simulink model "PV_MPPT_C2000_Algorithm"  (R2018b)
settings: Solver=FixedStepDiscrete  StartTime=0.0  StopTime=inf  FixedStep=1e-4  RelTol=1e-3  EnableMultiTasking=on
InitFcn:
  | IQ8 = 256;
  | IQ13 = 8192;
  | IQ15 = 32768;
  | IQ24 = 16777216;
  | 
  | InvFreq = 50;
  | 
  | Tdata = 0.05;
  | Tcontrol = 1e-4;
undefined symbols (not defined in the file): DiscIntNeverNeededParam, Down, GPTRIP1SEL, GPTRIP2SEL, TZ1, TZ2, Up
libraries: c2802xlib x8, simulink x4, c280xlib x3
settings Model: ExtModeTrigDuration=8  Creator=The MathWorks, Inc.  LastModifiedBy=jlesage
settings DataIOCC: LimitDataPoints=on  SaveFormat=Array  SaveOutput=off  SaveTime=off  SignalLoggingName=sigsOut
settings OptimizationCC: DefaultUnderspecifiedDataType=single  ExpressionDepthLimit=2147483647  InitFltsAndDblsToZero=on  LifeSpan=1  MaxStackSize=512
settings DebuggingCC: UnderspecifiedInitializationDetection=Classic  MergeDetectMultiDrivingBlocksExec=none  CheckExecutionContextPreStartOutputMsg=on  CheckExecutionContextRuntimeOutputMsg=on  SignalResolutionControl=TryResolveAllWithWarning  MultiTaskDSMMsg=warning  MultiTaskCondExecSysMsg=none  SigSpecEnsureSampleTimeMsg=none  FcnCallInpInsideContextMsg=warning  AllowSymbolicDim=off  StateNameClashWarn=warning  LibraryContextMissingDiagnostic=none  SFUnexpectedBacktrackingDiag=warning  SFNoUnconditionalDefaultTransitionDiag=warning  SFExecutionAtInitializationDiag=none
settings HardwareCC: ProdBitPerChar=16  ProdBitPerInt=16  ProdBitPerPointer=32  ProdBitPerSizeT=32  ProdBitPerPtrDiffT=32  ProdLargestAtomicInteger=Integer  ProdLargestAtomicFloat=None  ProdWordSize=16  ProdLongLongMode=on  ProdHWDeviceType=Texas Instruments->C2000  TargetBitPerChar=16  TargetBitPerInt=16  TargetBitPerPointer=16  TargetLargestAtomicInteger=Integer  TargetIntDivRoundTo=Zero  TargetEndianess=LittleEndian  TargetWordSize=16  TargetHWDeviceType=Texas Instruments->C2000  ProdEqTarget=off
settings ModelReferenceCC: UpdateModelReferenceTargets=IfOutOfDate  PropagateSignalLabelsOutOfModel=off
settings SFSimCC: SimUseLocalCustomCode=off
settings RTWCC: SystemTargetFile=ert.tlc  HardwareBoard=TI Piccolo F2803x  TemplateMakefile=ert_default_tmf  PostCodeGenCommand=; codertarget.postCodeGenHookCommand(h)  RTWUseLocalCustomCode=off  Toolchain=Texas Instruments Code Composer Studio (C2000)
settings CodeAppCC: IgnoreCustomStorageClasses=off  CustomSymbolStrType=$N$R$M  StateflowObjectComments=on  InternalIdentifier=Classic
settings ERTTargetCC: CodeReplacementLibrary=TI C28x  MultiwordLength=2048  ParMdlRefBuildCompliant=off  CompOptLevelCompliant=off  ConcurrentExecutionCompliant=off  SupportNonFinite=off  SupportComplex=off  CPPClassGenCompliant=off  ExtModeStaticAllocSize=2048  ConvertIfToSwitch=off  SuppressUnreachableDefaultCases=off
settings ConfigComp: CovMetricSettings=dw  CovHtmlReporting=on  CovSaveCumulativeToWorkspaceVar=on  CovSaveSingleToWorkspaceVar=on  CovExternalEMLEnable=off  CovSFcnEnable=off

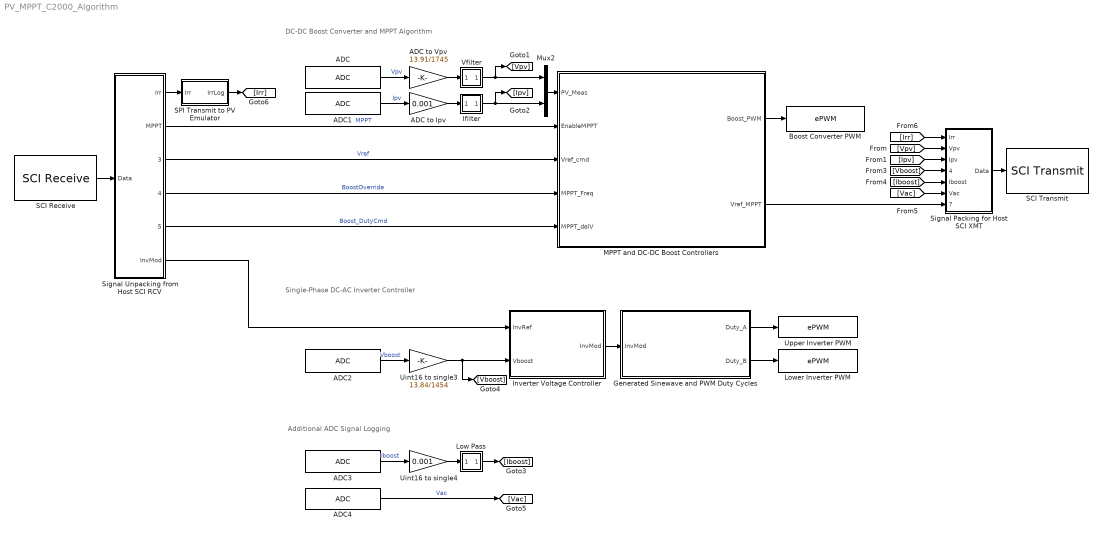
== system PV_MPPT_C2000_Algorithm ==
  note: Additional ADC Signal Logging
  note: Single-Phase DC-AC Inverter Controller
  note: DC-DC Boost Converter and MPPT Algorithm
  ADC : c2802xlib/ADC  ADCModule=1  samplingMode=Single sample mode  ADCResolution=12-bit (Single-ended input)  useSOC1=SOC0  useSOC2=SOC0_SOC1  SOCAcquisitionWindow=7  SOCTriggerSource=Software  SOCInterruptTrigger=No ADCINT  Ts=Tcontrol  dType=uint16  postInterrupt=off  interruptSel=ADCINT1  ADCINTContinuous=off  endma=off  chdma=1  blkParamProc=C2000  conv1=ADCINA1  conv2=ADCINA0 and ADCINB0  conv1_Type4=ADCIN0  conv2_Type4=ADCIN0 and ADCIN1
      settings: SourceProductName=Embedded Coder Support Package for Texas Instruments C2000 Processors
  ADC to Ipv : Gain  Gain=0.001  OutDataTypeStr=single
  ADC to Vpv : Gain  Gain=13.91/1745  OutDataTypeStr=single
  ADC1 : c2802xlib/ADC  ADCModule=1  samplingMode=Single sample mode  ADCResolution=12-bit (Single-ended input)  useSOC1=SOC1  useSOC2=SOC0_SOC1  SOCAcquisitionWindow=7  SOCTriggerSource=Software  SOCInterruptTrigger=No ADCINT  Ts=Tcontrol  dType=uint16  postInterrupt=off  interruptSel=ADCINT1  ADCINTContinuous=off  endma=off  chdma=1  blkParamProc=C2000  conv1=ADCINA0  conv2=ADCINA0 and ADCINB0  conv1_Type4=ADCIN0  conv2_Type4=ADCIN0 and ADCIN1
      settings: SourceProductName=Embedded Coder Support Package for Texas Instruments C2000 Processors
  ADC2 : c2802xlib/ADC  ADCModule=1  samplingMode=Single sample mode  ADCResolution=12-bit (Single-ended input)  useSOC1=SOC2  useSOC2=SOC0_SOC1  SOCAcquisitionWindow=7  SOCTriggerSource=Software  SOCInterruptTrigger=No ADCINT  Ts=Tcontrol  dType=uint16  postInterrupt=off  interruptSel=ADCINT1  ADCINTContinuous=off  endma=off  chdma=1  blkParamProc=C2000  conv1=ADCINA2  conv2=ADCINA0 and ADCINB0  conv1_Type4=ADCIN0  conv2_Type4=ADCIN0 and ADCIN1
      settings: SourceProductName=Embedded Coder Support Package for Texas Instruments C2000 Processors
  ADC3 : c2802xlib/ADC  ADCModule=1  samplingMode=Single sample mode  ADCResolution=12-bit (Single-ended input)  useSOC1=SOC3  useSOC2=SOC0_SOC1  SOCAcquisitionWindow=7  SOCTriggerSource=Software  SOCInterruptTrigger=No ADCINT  Ts=Tcontrol  dType=uint16  postInterrupt=off  interruptSel=ADCINT1  ADCINTContinuous=off  endma=off  chdma=1  blkParamProc=C2000  conv1=ADCINB6  conv2=ADCINA0 and ADCINB0  conv1_Type4=ADCIN0  conv2_Type4=ADCIN0 and ADCIN1
      settings: SourceProductName=Embedded Coder Support Package for Texas Instruments C2000 Processors
  ADC4 : c2802xlib/ADC  ADCModule=1  samplingMode=Single sample mode  ADCResolution=12-bit (Single-ended input)  useSOC1=SOC4  useSOC2=SOC0_SOC1  SOCAcquisitionWindow=7  SOCTriggerSource=Software  SOCInterruptTrigger=No ADCINT  Ts=Tcontrol  dType=uint16  postInterrupt=off  interruptSel=ADCINT1  ADCINTContinuous=off  endma=off  chdma=1  blkParamProc=C2000  conv1=ADCINA7  conv2=ADCINA0 and ADCINB0  conv1_Type4=ADCIN0  conv2_Type4=ADCIN0 and ADCIN1
      settings: SourceProductName=Embedded Coder Support Package for Texas Instruments C2000 Processors
  Boost Converter PWM : c2802xlib/ePWM  useModule=ePWM3  ePWMxLINKTBPRD=Not Linked  periodUnits=Clock cycles  timerSource=Specify via dialog  timerPeriod_clk=1500  timerPeriod_sec=0.0001  tbshadow=Counter equals to zero  countingMode=Up-Down  phaseActiveEnable=Set counter to phase value specified via dialog  phaseDirection=Count up after sync  phaseActive=4  synchronizationEnable=off  dcaevt1Sync=off  dcbevt1Sync=off  synchronizationOption=Disable  clockPrescale=1  HSclockPrescale=1  enswap=off  ePWMxAStatus=on  ePWMxAactionLogic1=Do nothing  ePWMxAactionLogic2=Do nothing  ePWMxAactionLogic3=Set  ePWMxAactionLogic4=Clear  ePWMxAactionLogic5=Do nothing  ePWMxAactionLogic6=Do nothing  ePWMxALoadMode=Load on counter equals to zero (CTR=Zero)  ePWMxACSFenable=off  ePWMxACSFvalue=Forcing disable  ePWMxASFreload=Zero  ePWMxBStatus=off  ePWMxBactionLogic1=Do nothing  ePWMxBactionLogic2=Do nothing  ePWMxBactionLogic3=Do nothing  ePWMxBactionLogic4=Do nothing  ePWMxBactionLogic5=Do nothing  ePWMxBactionLogic6=Do nothing  ePWMxBLoadMode=Load on counter equals to zero (CTR=Zero)  ePWMxBCSFenable=off  ePWMxBCSFvalue=Forcing disable  ePWMxBSFreload=Zero  ePWNxBOutWay=off  ePWMxLINKCMPA=Not Linked  CMPAUnits=Clock cycles  CMPASource=Input port  CMPAValue_per=0  CMPAValue_clk=0  enCMPAshadow=Counter equals to zero  ePWMxLINKCMPB=Not Linked  CMPBUnits=Clock cycles  CMPBSource=Specify via dialog  CMPBValue_per=50  CMPBValue_clk=0  enCMPBshadow=Counter equals to zero  ePWMxLINKCMPC=Not Linked  CMPCUnits=Clock cycles  CMPCSource=Specify via dialog  CMPCValue_per=50  CMPCValue_clk=32000  enCMPCshadow=Counter equals to zero  ePWMxLINKCMPD=Not Linked  CMPDUnits=Clock cycles  CMPDSource=Specify via dialog  CMPDValue_per=50  CMPDValue_clk=32000  enCMPDshadow=Counter equals to zero  enableDBePWMxA=on  enableDBePWMxB=on  enhalfcycle=off  DBpolarity=Active high (AH)  DBedgeDelay=Positive  DBSource_ePWMxA=ePWMxA  DBSource_ePWMxB=ePWMxA  DBperiodSource=Specify via dialog  REDperiod=0  FEDperiod=30  adcstartModuleA=on  adcrequestEventA=Second event  adcstartEventA=Counter is incrementing and equals to the compare B register (CTRU=CMPB)  adcstartEventA_type2=Digital Compare Module A Event 1 start of conversion (DCAEVT1.soc)  adcstartModuleB=off  adcrequestEventB=First event  adcstartEventB=Counter equals to zero (CTR=Zero)  adcstartEventB_type2=Counter equals to zero (CTR=Zero)  intEn=on  intPrd=Second event  intSel=Counter equals to period (CTR=PRD)  intSel_type2=Counter equals to zero (CTR=Zero)  hrpe=off  enHRPWM=off  HRPWM_LoadMode=Counter equals to period (CTR=PRD)  HRPWM_CTLMode=Duty or Period control mode  HRPWM_EDGMode=Falling edge  hrpeb=off  enHRPWMB=off  HRPWM_LoadModeB=Counter equals to zero (CTR=ZERO)  HRPWM_CTLModeB=Duty or Period control mode  HRPWM_EDGModeB=Both edge  enSFO=off  enautoconv=off  chopperEnable=off  chopperFrequency=1  chopperFirstwidth=1  chopperDuty=12.5%  tripZonesource=Specify via dialog  tzselOSHT1=off  tzselOSHT2=off  tzselOSHT3=off  tzselOSHDCAEV1=on  tzselOSHDCBEV1=off  tzselCBC1=off  tzselCBC2=off  tzselCBC3=off  tzselCBCDCAEV2=on  tzselCBCDCBEV2=off  tzselOSHT4=off  tzselOSHT5=off  tzselOSHT6=off  tzselCBC4=off  tzselCBC5=off  tzselCBC6=off  enTzOstIntr=off  enTzCbcIntr=off  enTzDCAEVT1Intr=off  enTzDCAEVT2Intr=off  enTzDCBEVT1Intr=off  enTzDCBEVT2Intr=off  ePWMxAforced=Low  ePWMxBforced=No action  DCAEVT1forced=No action  DCBEVT1forced=No action  DCAEVT2forced=No action  DCBEVT2forced=No action  dcah=COMP1OUT input  dcal=Trip Zone 2 input (TZ2)  dcbh=Trip Zone 1 input (TZ1)  dcbl=Trip Zone 2 input (TZ2)  dcah_type2=GPTRIP1SEL/(TZ1)  dcal_type2=GPTRIP2SEL/(TZ2)  dcbh_type2=GPTRIP1SEL/(TZ1)  dcbl_type2=GPTRIP2SEL/(TZ2)  gendcaevt1=DCAH=high and DCAL=don't care  gendcaevt2=Event disabled  gendcbevt1=Event disabled  gendcbevt2=Event disabled  dcaevt1src=DCAEVT1 with async  dcaevt2src=DCAEVT2 with sync  dcbevt1src=DCBEVT1 with sync  dcbevt2src=DCBEVT2 with sync  pulsesel=Counter equals to zero (CTR=Zero)  blankinv=off  blankoffset=0  blankwidth=0  evsrcsel=Filtered version of DCAEVT1 (DCAEVT1FILT)  encape=off  PwmType=C2000
      settings: SourceProductName=Embedded Coder Support Package for Texas Instruments C2000 Processors
  Generated Sinewave and PWM Duty Cycles : Subsystem
  Ifilter : Subsystem  mask{Tf=0.01}
      mask prompts: Tf "Filter Time Constant"
  Inverter Voltage Controller : Subsystem
  Low Pass : Subsystem  mask{Tf=0.01}
      mask prompts: Tf "Filter Time Constant"
  Lower Inverter PWM : c2802xlib/ePWM  useModule=ePWM2  ePWMxLINKTBPRD=Not Linked  periodUnits=Clock cycles  timerSource=Specify via dialog  timerPeriod_clk=1500  timerPeriod_sec=0.0001  tbshadow=Counter equals to zero  countingMode=Up-Down  phaseActiveEnable=Set counter to phase value specified via dialog  phaseDirection=Count up after sync  phaseActive=2  synchronizationEnable=off  dcaevt1Sync=off  dcbevt1Sync=off  synchronizationOption=Counter equals to zero (CTR=Zero)  clockPrescale=1  HSclockPrescale=1  enswap=off  ePWMxAStatus=on  ePWMxAactionLogic1=Do nothing  ePWMxAactionLogic2=Do nothing  ePWMxAactionLogic3=Clear  ePWMxAactionLogic4=Set  ePWMxAactionLogic5=Do nothing  ePWMxAactionLogic6=Do nothing  ePWMxALoadMode=Load on counter equals to period (CTR=PRD)  ePWMxACSFenable=off  ePWMxACSFvalue=Forcing disable  ePWMxASFreload=Zero  ePWMxBStatus=off  ePWMxBactionLogic1=Do nothing  ePWMxBactionLogic2=Do nothing  ePWMxBactionLogic3=Do nothing  ePWMxBactionLogic4=Do nothing  ePWMxBactionLogic5=Do nothing  ePWMxBactionLogic6=Do nothing  ePWMxBLoadMode=Load on counter equals to zero (CTR=Zero)  ePWMxBCSFenable=off  ePWMxBCSFvalue=Forcing disable  ePWMxBSFreload=Zero  ePWNxBOutWay=on  ePWMxLINKCMPA=Not Linked  CMPAUnits=Clock cycles  CMPASource=Input port  CMPAValue_per=0  CMPAValue_clk=750  enCMPAshadow=Counter equals to zero  ePWMxLINKCMPB=Not Linked  CMPBUnits=Clock cycles  CMPBSource=Specify via dialog  CMPBValue_per=50  CMPBValue_clk=0  enCMPBshadow=Counter equals to zero  ePWMxLINKCMPC=Not Linked  CMPCUnits=Clock cycles  CMPCSource=Specify via dialog  CMPCValue_per=50  CMPCValue_clk=32000  enCMPCshadow=Counter equals to zero  ePWMxLINKCMPD=Not Linked  CMPDUnits=Clock cycles  CMPDSource=Specify via dialog  CMPDValue_per=50  CMPDValue_clk=32000  enCMPDshadow=Counter equals to zero  enableDBePWMxA=on  enableDBePWMxB=on  enhalfcycle=off  DBpolarity=Active high complementary (AHC)  DBedgeDelay=Positive  DBSource_ePWMxA=ePWMxA  DBSource_ePWMxB=ePWMxB  DBperiodSource=Specify via dialog  REDperiod=20  FEDperiod=20  adcstartModuleA=on  adcrequestEventA=First event  adcstartEventA=Counter equals to zero (CTR=Zero)  adcstartEventA_type2=Digital Compare Module A Event 1 start of conversion (DCAEVT1.soc)  adcstartModuleB=off  adcrequestEventB=First event  adcstartEventB=Counter equals to zero (CTR=Zero)  adcstartEventB_type2=Counter equals to zero (CTR=Zero)  intEn=off  intPrd=First event  intSel=Counter equals to period (CTR=PRD)  intSel_type2=Counter equals to zero (CTR=Zero)  hrpe=off  enHRPWM=off  HRPWM_LoadMode=Counter equals to period (CTR=PRD)  HRPWM_CTLMode=Duty or Period control mode  HRPWM_EDGMode=Falling edge  hrpeb=off  enHRPWMB=off  HRPWM_LoadModeB=Counter equals to zero (CTR=ZERO)  HRPWM_CTLModeB=Duty or Period control mode  HRPWM_EDGModeB=Both edge  enSFO=off  enautoconv=off  chopperEnable=off  chopperFrequency=1  chopperFirstwidth=1  chopperDuty=12.5%  tripZonesource=Specify via dialog  tzselOSHT1=off  tzselOSHT2=off  tzselOSHT3=off  tzselOSHDCAEV1=on  tzselOSHDCBEV1=off  tzselCBC1=off  tzselCBC2=off  tzselCBC3=off  tzselCBCDCAEV2=on  tzselCBCDCBEV2=off  tzselOSHT4=off  tzselOSHT5=off  tzselOSHT6=off  tzselCBC4=off  tzselCBC5=off  tzselCBC6=off  enTzOstIntr=off  enTzCbcIntr=off  enTzDCAEVT1Intr=off  enTzDCAEVT2Intr=off  enTzDCBEVT1Intr=off  enTzDCBEVT2Intr=off  ePWMxAforced=Low  ePWMxBforced=No action  DCAEVT1forced=No action  DCBEVT1forced=No action  DCAEVT2forced=No action  DCBEVT2forced=No action  dcah=COMP1OUT input  dcal=Trip Zone 2 input (TZ2)  dcbh=Trip Zone 1 input (TZ1)  dcbl=Trip Zone 2 input (TZ2)  dcah_type2=GPTRIP1SEL/(TZ1)  dcal_type2=GPTRIP2SEL/(TZ2)  dcbh_type2=GPTRIP1SEL/(TZ1)  dcbl_type2=GPTRIP2SEL/(TZ2)  gendcaevt1=DCAH=high and DCAL=don't care  gendcaevt2=Event disabled  gendcbevt1=Event disabled  gendcbevt2=Event disabled  dcaevt1src=DCAEVT1 with async  dcaevt2src=DCAEVT2 with sync  dcbevt1src=DCBEVT1 with sync  dcbevt2src=DCBEVT2 with sync  pulsesel=Counter equals to zero (CTR=Zero)  blankinv=off  blankoffset=0  blankwidth=0  evsrcsel=Filtered version of DCAEVT1 (DCAEVT1FILT)  encape=off  PwmType=C2000
      settings: SourceProductName=Embedded Coder Support Package for Texas Instruments C2000 Processors
  MPPT and DC-DC Boost Controllers : Subsystem
  Mux2 : Mux  Inputs=2
  SCI Receive : c280xlib/SCI Receive  sciModule=A  dataHead='B'  dataTail='T'  dataType=uint16  dataDim=6  initValue=[0.1*IQ13 0.1*IQ13 25*IQ8 0.1*IQ13 0 3*IQ8]  errOption=Output the last received value  errValue=0.5*IQ13  sampleTime=Tdata  outputStatus=off  postInterrupt=off  numFifo=0
      settings: SourceProductName=Embedded Coder Support Package for Texas Instruments C2000 Processors  SourceProductBaseCode=TIC2000
  SCI Transmit : c280xlib/SCI Transmit  sciModule=A  dataHead='S'  dataTail='E'  postInterrupt=off  numFifo=0
      settings: SourceProductName=Embedded Coder Support Package for Texas Instruments C2000 Processors
  SPI Transmit to PV Emulator : Subsystem
  Signal Packing for Host SCI XMT : Subsystem
  Signal Unpacking from Host SCI RCV : Subsystem
  Uint16 to single3 : Gain  Gain=13.84/1454  OutDataTypeStr=single
  Uint16 to single4 : Gain  Gain=0.001  OutDataTypeStr=single
  Upper Inverter PWM : c2802xlib/ePWM  useModule=ePWM1  ePWMxLINKTBPRD=Not Linked  periodUnits=Clock cycles  timerSource=Specify via dialog  timerPeriod_clk=1500  timerPeriod_sec=0.0001  tbshadow=Counter equals to zero  countingMode=Up-Down  phaseActiveEnable=Disable  phaseDirection=Count down after sync  phaseActive=750  synchronizationEnable=off  dcaevt1Sync=off  dcbevt1Sync=off  synchronizationOption=Counter equals to zero (CTR=Zero)  clockPrescale=1  HSclockPrescale=1  enswap=off  ePWMxAStatus=on  ePWMxAactionLogic1=Do nothing  ePWMxAactionLogic2=Do nothing  ePWMxAactionLogic3=Clear  ePWMxAactionLogic4=Set  ePWMxAactionLogic5=Do nothing  ePWMxAactionLogic6=Do nothing  ePWMxALoadMode=Load on counter equals to zero (CTR=Zero)  ePWMxACSFenable=off  ePWMxACSFvalue=Forcing disable  ePWMxASFreload=Zero  ePWMxBStatus=off  ePWMxBactionLogic1=Do nothing  ePWMxBactionLogic2=Do nothing  ePWMxBactionLogic3=Do nothing  ePWMxBactionLogic4=Do nothing  ePWMxBactionLogic5=Do nothing  ePWMxBactionLogic6=Do nothing  ePWMxBLoadMode=Load on counter equals to zero (CTR=Zero)  ePWMxBCSFenable=off  ePWMxBCSFvalue=Forcing disable  ePWMxBSFreload=Zero  ePWNxBOutWay=on  ePWMxLINKCMPA=Not Linked  CMPAUnits=Clock cycles  CMPASource=Input port  CMPAValue_per=0  CMPAValue_clk=750  enCMPAshadow=Counter equals to zero  ePWMxLINKCMPB=Not Linked  CMPBUnits=Clock cycles  CMPBSource=Specify via dialog  CMPBValue_per=50  CMPBValue_clk=0  enCMPBshadow=Counter equals to zero  ePWMxLINKCMPC=Not Linked  CMPCUnits=Clock cycles  CMPCSource=Specify via dialog  CMPCValue_per=50  CMPCValue_clk=32000  enCMPCshadow=Counter equals to zero  ePWMxLINKCMPD=Not Linked  CMPDUnits=Clock cycles  CMPDSource=Specify via dialog  CMPDValue_per=50  CMPDValue_clk=32000  enCMPDshadow=Counter equals to zero  enableDBePWMxA=on  enableDBePWMxB=on  enhalfcycle=off  DBpolarity=Active high complementary (AHC)  DBedgeDelay=Positive  DBSource_ePWMxA=ePWMxA  DBSource_ePWMxB=ePWMxB  DBperiodSource=Specify via dialog  REDperiod=20  FEDperiod=20  adcstartModuleA=on  adcrequestEventA=First event  adcstartEventA=Counter equals to zero (CTR=Zero)  adcstartEventA_type2=Digital Compare Module A Event 1 start of conversion (DCAEVT1.soc)  adcstartModuleB=off  adcrequestEventB=First event  adcstartEventB=Counter equals to zero (CTR=Zero)  adcstartEventB_type2=Counter equals to zero (CTR=Zero)  intEn=off  intPrd=First event  intSel=Counter equals to period (CTR=PRD)  intSel_type2=Counter equals to zero (CTR=Zero)  hrpe=off  enHRPWM=off  HRPWM_LoadMode=Counter equals to period (CTR=PRD)  HRPWM_CTLMode=Duty or Period control mode  HRPWM_EDGMode=Falling edge  hrpeb=off  enHRPWMB=off  HRPWM_LoadModeB=Counter equals to zero (CTR=ZERO)  HRPWM_CTLModeB=Duty or Period control mode  HRPWM_EDGModeB=Both edge  enSFO=off  enautoconv=off  chopperEnable=off  chopperFrequency=1  chopperFirstwidth=1  chopperDuty=12.5%  tripZonesource=Specify via dialog  tzselOSHT1=off  tzselOSHT2=off  tzselOSHT3=off  tzselOSHDCAEV1=on  tzselOSHDCBEV1=off  tzselCBC1=off  tzselCBC2=off  tzselCBC3=off  tzselCBCDCAEV2=on  tzselCBCDCBEV2=off  tzselOSHT4=off  tzselOSHT5=off  tzselOSHT6=off  tzselCBC4=off  tzselCBC5=off  tzselCBC6=off  enTzOstIntr=off  enTzCbcIntr=off  enTzDCAEVT1Intr=off  enTzDCAEVT2Intr=off  enTzDCBEVT1Intr=off  enTzDCBEVT2Intr=off  ePWMxAforced=Low  ePWMxBforced=No action  DCAEVT1forced=No action  DCBEVT1forced=No action  DCAEVT2forced=No action  DCBEVT2forced=No action  dcah=COMP1OUT input  dcal=Trip Zone 2 input (TZ2)  dcbh=Trip Zone 1 input (TZ1)  dcbl=Trip Zone 2 input (TZ2)  dcah_type2=GPTRIP1SEL/(TZ1)  dcal_type2=GPTRIP2SEL/(TZ2)  dcbh_type2=GPTRIP1SEL/(TZ1)  dcbl_type2=GPTRIP2SEL/(TZ2)  gendcaevt1=DCAH=high and DCAL=don't care  gendcaevt2=Event disabled  gendcbevt1=Event disabled  gendcbevt2=Event disabled  dcaevt1src=DCAEVT1 with async  dcaevt2src=DCAEVT2 with sync  dcbevt1src=DCBEVT1 with sync  dcbevt2src=DCBEVT2 with sync  pulsesel=Counter equals to zero (CTR=Zero)  blankinv=off  blankoffset=0  blankwidth=0  evsrcsel=Filtered version of DCAEVT1 (DCAEVT1FILT)  encape=off  PwmType=C2000
      settings: SourceProductName=Embedded Coder Support Package for Texas Instruments C2000 Processors
  Vfilter : Subsystem  mask{Tf=0.01}
      mask prompts: Tf "Filter Time Constant"
  wires:
  ADC/1 -> ADC to Vpv/1  "Vpv"
  ADC1/1 -> ADC to Ipv/1  "Ipv"
  ADC2/1 -> Uint16 to single3/1  "Vboost"
  ADC3/1 -> Uint16 to single4/1  "Iboost"
  Generated Sinewave and PWM Duty Cycles/1(Duty_A) -> Upper Inverter PWM/1
  Generated Sinewave and PWM Duty Cycles/2(Duty_B) -> Lower Inverter PWM/1
  ADC to Vpv/1 -> Vfilter/1(u)
  ADC to Ipv/1 -> Ifilter/1(u)
  Uint16 to single4/1 -> Low Pass/1(u)
  ADC4/1 -> [Vac]  "Vac"
  MPPT and DC-DC Boost Controllers/1(Boost_PWM) -> Boost Converter PWM/1
  Mux2/1 -> MPPT and DC-DC Boost Controllers/1(PV_Meas)
  [Irr] -> Signal Packing for Host SCI XMT/1(Irr)
  [Vpv] -> Signal Packing for Host SCI XMT/2(Vpv)
  [Ipv] -> Signal Packing for Host SCI XMT/3(Ipv)
  [Vboost] -> Signal Packing for Host SCI XMT/4(Vboost)
  [Iboost] -> Signal Packing for Host SCI XMT/5(Iboost)
  [Vac] -> Signal Packing for Host SCI XMT/6(Vac)
  MPPT and DC-DC Boost Controllers/2(Vref_MPPT) -> Signal Packing for Host SCI XMT/7(Dboost)
  Signal Packing for Host SCI XMT/1(Data) -> SCI Transmit/1
  Signal Unpacking from Host SCI RCV/5(MPPT_Vinc) -> MPPT and DC-DC Boost Controllers/5(MPPT_delV)  "Boost_DutyCmd"
  Signal Unpacking from Host SCI RCV/4(MPPT_Freq) -> MPPT and DC-DC Boost Controllers/4(MPPT_Freq)  "BoostOverride"
  Signal Unpacking from Host SCI RCV/2(MPPT) -> MPPT and DC-DC Boost Controllers/2(EnableMPPT)  "MPPT"
  Signal Unpacking from Host SCI RCV/3(Vref_cmd) -> MPPT and DC-DC Boost Controllers/3(Vref_cmd)  "Vref"
  Uint16 to single3/1 -> [Vboost], Inverter Voltage Controller/2(Vboost)
  Signal Unpacking from Host SCI RCV/6(InvMod) -> Inverter Voltage Controller/1(InvRef)
  Inverter Voltage Controller/1(InvMod) -> Generated Sinewave and PWM Duty Cycles/1(InvMod)
  Signal Unpacking from Host SCI RCV/1(Irr) -> SPI Transmit to PV Emulator/1(Irr)
  SCI Receive/1 -> Signal Unpacking from Host SCI RCV/1(Data)
  SPI Transmit to PV Emulator/1(IrrLog) -> [Irr]
  Vfilter/1(y) -> Mux2/1, [Vpv]
  Ifilter/1(y) -> Mux2/2, [Ipv]
  Low Pass/1(y) -> [Iboost]

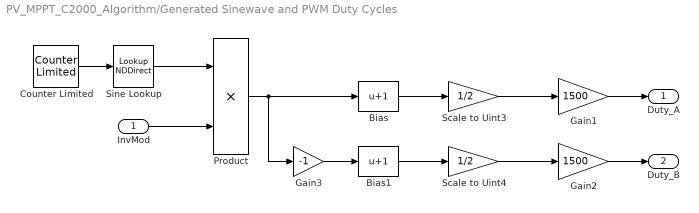
== system PV_MPPT_C2000_Algorithm/Generated Sinewave and PWM Duty Cycles ==
  InvMod : Inport
  Bias : Bias  Bias=1
  Bias1 : Bias  Bias=1
  Counter Limited : simulink/Sources/Counter Limited  uplimit=floor(1/(InvFreq*Tcontrol))  tsamp=Tcontrol
  Gain1 : Gain  Gain=1500  ParamDataTypeStr=uint16  OutDataTypeStr=uint16  RndMeth=Simplest
  Gain2 : Gain  Gain=1500  ParamDataTypeStr=uint16  OutDataTypeStr=uint16  RndMeth=Simplest
  Gain3 : Gain  Gain=-1
  Product : Product
  Scale to Uint3 : Gain  Gain=1/2  OutDataTypeStr=single
  Scale to Uint4 : Gain  Gain=1/2  OutDataTypeStr=single
  Sine Lookup : LookupNDDirect  NumberOfTableDimensions=1  Table=sin( 2*pi * (0:floor(1/(InvFreq*Tcontrol)))/floor(1/(InvFreq*Tcontrol))+90/180)'  TableDataTypeStr=single
  Duty_A : Outport
  Duty_B : Outport  Port=2
  wires:
  Bias/1 -> Scale to Uint3/1
  Scale to Uint4/1 -> Gain2/1
  InvMod/1 -> Product/2
  Bias1/1 -> Scale to Uint4/1
  Scale to Uint3/1 -> Gain1/1
  Product/1 -> Gain3/1, Bias/1
  Gain3/1 -> Bias1/1
  Sine Lookup/1 -> Product/1
  Counter Limited/1 -> Sine Lookup/1
  Gain1/1 -> Duty_A/1
  Gain2/1 -> Duty_B/1

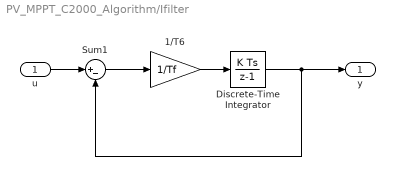
== system PV_MPPT_C2000_Algorithm/Ifilter ==
  u : Inport
  1/T6 : Gain  Gain=1/Tf
  Discrete-Time Integrator : DiscreteIntegrator  SampleTime=Tcontrol  ICPrevOutput=DiscIntNeverNeededParam  ICPrevScaledInput=DiscIntNeverNeededParam
  Sum1 : Sum  Inputs=|+-
  y : Outport
  wires:
  Sum1/1 -> 1/T6/1
  Discrete-Time Integrator/1 -> Sum1/2, y/1
  u/1 -> Sum1/1
  1/T6/1 -> Discrete-Time Integrator/1

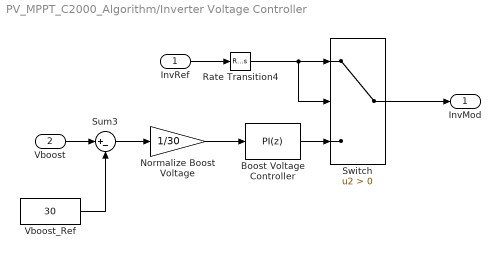
== system PV_MPPT_C2000_Algorithm/Inverter Voltage Controller ==
  InvRef : Inport
  Vboost : Inport  Port=2
  Boost Voltage Controller : simulink/Continuous/PID Controller  Controller=PI  TimeDomain=Discrete-time  SampleTime=Tcontrol  IntegratorMethod=Forward Euler  FilterMethod=Forward Euler  Form=Parallel  UseFilter=on  ControllerParametersSource=internal  P=3  I=250  D=0  N=100  InitialConditionSource=internal  InitialConditionForIntegrator=1  InitialConditionForFilter=0  ExternalReset=none  LimitOutput=on  UpperSaturationLimit=1  LowerSaturationLimit=0  LinearizeAsGain=on  AntiWindupMode=clamping  Kb=1  TrackingMode=off  Kt=1  PParamMin=[]  PParamMax=[]  IParamMin=[]  IParamMax=[]  DParamMin=[]  DParamMax=[]  NParamMin=[]  NParamMax=[]  KbParamMin=[]  KbParamMax=[]  KtParamMin=[]  KtParamMax=[]  POutMin=[]  POutMax=[]  IOutMin=[]  IOutMax=[]  DOutMin=[]  DOutMax=[]  NOutMin=[]  NOutMax=[]  KbOutMin=[]  KbOutMax=[]  KtOutMin=[]  KtOutMax=[]  IntegratorOutMin=[]  IntegratorOutMax=[]  FilterOutMin=[]  FilterOutMax=[]  SumOutMin=[]  SumOutMax=[]  SumI1OutMin=[]  SumI1OutMax=[]  SumI2OutMin=[]  SumI2OutMax=[]  SumI3OutMin=[]  SumI3OutMax=[]  SumDOutMin=[]  SumDOutMax=[]  SaturationOutMin=[]  SaturationOutMax=[]  IntegratorContinuousStateAttributes=''  IntegratorStateMustResolveToSignalObject=off  IntegratorRTWStateStorageClass=Auto  FilterContinuousStateAttributes=''  FilterStateMustResolveToSignalObject=off  FilterRTWStateStorageClass=Auto  DifferentiatorICPrevScaledInput=0  DifferentiatorOutMin=[]  DifferentiatorOutMax=[]  InitialConditionSetting=State (most efficient)  FilterDiffOutCoefMin=[]  FilterDiffOutCoefMax=[]  SumDenOutMin=[]  SumDenOutMax=[]  SumNumOutMin=[]  SumNumOutMax=[]  ReciprocalOutMin=[]  ReciprocalOutMax=[]  DivideOutMin=[]  DivideOutMax=[]  TunerSelectOption=Transfer Function Based (PID Tuner App)
  Normalize Boost Voltage : Gain  Gain=1/30
  Rate Transition4 : RateTransition  Integrity=off  Deterministic=off  InitialCondition=0.1*IQ24  OutPortSampleTime=Tcontrol
  Sum3 : Sum  Inputs=|+-
  Switch : Switch  Criteria=u2 > Threshold
  Vboost_Ref : Constant  Value=30  OutDataTypeStr=single
  InvMod : Outport
  wires:
  InvRef/1 -> Rate Transition4/1
  Rate Transition4/1 -> Switch/2, Switch/1
  Vboost_Ref/1 -> Sum3/2
  Sum3/1 -> Normalize Boost Voltage/1
  Normalize Boost Voltage/1 -> Boost Voltage Controller/1
  Switch/1 -> InvMod/1
  Boost Voltage Controller/1 -> Switch/3
  Vboost/1 -> Sum3/1

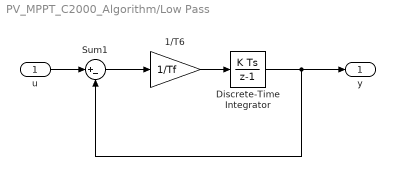
== system PV_MPPT_C2000_Algorithm/Low Pass ==
  u : Inport
  1/T6 : Gain  Gain=1/Tf
  Discrete-Time Integrator : DiscreteIntegrator  SampleTime=Tcontrol  ICPrevOutput=DiscIntNeverNeededParam  ICPrevScaledInput=DiscIntNeverNeededParam
  Sum1 : Sum  Inputs=|+-
  y : Outport
  wires:
  1/T6/1 -> Discrete-Time Integrator/1
  u/1 -> Sum1/1
  Discrete-Time Integrator/1 -> y/1, Sum1/2
  Sum1/1 -> 1/T6/1

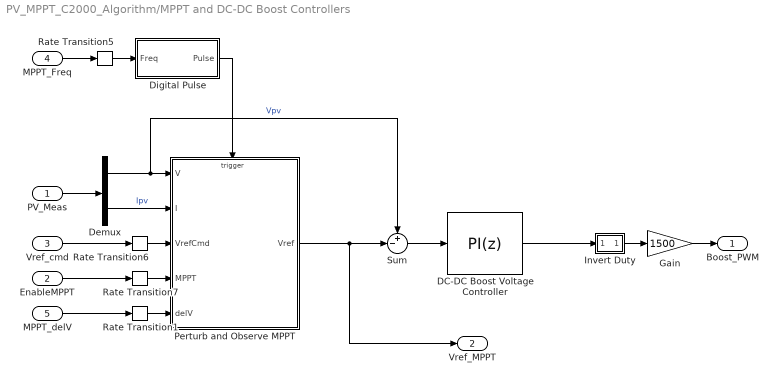
== system PV_MPPT_C2000_Algorithm/MPPT and DC-DC Boost Controllers ==
  PV_Meas : Inport
  EnableMPPT : Inport  Port=2
  Vref_cmd : Inport  Port=3
  MPPT_Freq : Inport  Port=4
  MPPT_delV : Inport  Port=5
  DC-DC Boost Voltage Controller : simulink/Continuous/PID Controller  Controller=PI  TimeDomain=Discrete-time  SampleTime=Tcontrol  IntegratorMethod=Forward Euler  FilterMethod=Forward Euler  Form=Parallel  UseFilter=on  ControllerParametersSource=internal  P=0.015  I=2.5  D=0  N=100  InitialConditionSource=internal  InitialConditionForIntegrator=0  InitialConditionForFilter=0  ExternalReset=none  LimitOutput=on  UpperSaturationLimit=0.9  LowerSaturationLimit=0  LinearizeAsGain=on  AntiWindupMode=clamping  Kb=1  TrackingMode=off  Kt=1  PParamMin=[]  PParamMax=[]  IParamMin=[]  IParamMax=[]  DParamMin=[]  DParamMax=[]  NParamMin=[]  NParamMax=[]  KbParamMin=[]  KbParamMax=[]  KtParamMin=[]  KtParamMax=[]  POutMin=[]  POutMax=[]  IOutMin=[]  IOutMax=[]  DOutMin=[]  DOutMax=[]  NOutMin=[]  NOutMax=[]  KbOutMin=[]  KbOutMax=[]  KtOutMin=[]  KtOutMax=[]  IntegratorOutMin=[]  IntegratorOutMax=[]  FilterOutMin=[]  FilterOutMax=[]  SumOutMin=[]  SumOutMax=[]  SumI1OutMin=[]  SumI1OutMax=[]  SumI2OutMin=[]  SumI2OutMax=[]  SumI3OutMin=[]  SumI3OutMax=[]  SumDOutMin=[]  SumDOutMax=[]  SaturationOutMin=[]  SaturationOutMax=[]  IntegratorContinuousStateAttributes=''  IntegratorStateMustResolveToSignalObject=off  IntegratorRTWStateStorageClass=Auto  FilterContinuousStateAttributes=''  FilterStateMustResolveToSignalObject=off  FilterRTWStateStorageClass=Auto  DifferentiatorICPrevScaledInput=0  DifferentiatorOutMin=[]  DifferentiatorOutMax=[]  InitialConditionSetting=State (most efficient)  FilterDiffOutCoefMin=[]  FilterDiffOutCoefMax=[]  SumDenOutMin=[]  SumDenOutMax=[]  SumNumOutMin=[]  SumNumOutMax=[]  ReciprocalOutMin=[]  ReciprocalOutMax=[]  DivideOutMin=[]  DivideOutMax=[]  TunerSelectOption=Transfer Function Based (PID Tuner App)
  Demux : Demux  Outputs=2
  Digital Pulse : Subsystem  mask{Ts=Tcontrol, Duty=0.5}
      mask prompts: Ts "Sample Rate [s]"; Duty "Duty Cycle [0-1]"
  Gain : Gain  Gain=1500  OutDataTypeStr=uint16  RndMeth=Simplest
  Invert Duty : Subsystem
  Perturb and Observe MPPT : Stateflow chart  TreatAsAtomicUnit=on  SystemSampleTime=Tdata
  Rate Transition1 : RateTransition  InitialCondition=single(0.1)  OutPortSampleTime=Tcontrol
  Rate Transition5 : RateTransition  InitialCondition=single(25)  OutPortSampleTime=Tcontrol
  Rate Transition6 : RateTransition  InitialCondition=single(3)  OutPortSampleTime=Tcontrol
  Rate Transition7 : RateTransition  InitialCondition=single(0)  OutPortSampleTime=Tcontrol
  Sum : Sum  Inputs=+-|
  Boost_PWM : Outport
  Vref_MPPT : Outport  Port=2
  wires:
  Gain/1 -> Boost_PWM/1
  Invert Duty/1(D) -> Gain/1
  EnableMPPT/1 -> Rate Transition7/1
  Sum/1 -> DC-DC Boost Voltage Controller/1
  Demux/2 -> Perturb and Observe MPPT/2(I)  "Ipv"
  Demux/1 -> Perturb and Observe MPPT/1(V), Sum/1  "Vpv"
  PV_Meas/1 -> Demux/1
  Perturb and Observe MPPT/1(Vref) -> Sum/2, Vref_MPPT/1
  Vref_cmd/1 -> Rate Transition6/1
  MPPT_delV/1 -> Rate Transition1/1
  Rate Transition1/1 -> Perturb and Observe MPPT/5(delV)
  Digital Pulse/1(Pulse) -> Perturb and Observe MPPT/Trigger
  DC-DC Boost Voltage Controller/1 -> Invert Duty/1(u)
  Rate Transition5/1 -> Digital Pulse/1(Freq)
  MPPT_Freq/1 -> Rate Transition5/1
  Rate Transition6/1 -> Perturb and Observe MPPT/3(VrefCmd)
  Rate Transition7/1 -> Perturb and Observe MPPT/4(MPPT)

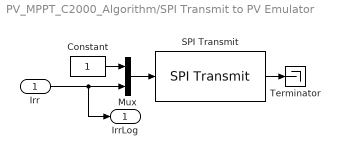
== system PV_MPPT_C2000_Algorithm/SPI Transmit to PV Emulator ==
  Irr : Inport
  Constant : Constant  OutDataTypeStr=uint16
  Mux : Mux  Inputs=2
  SPI Transmit : c280xlib/SPI Transmit  SPISelect=SPI_B  ClockPolarity=Rising_edge  ClockPhase=No_delay  SPIModule=uint32(0)  Mode=Master  BusSpeed=uint32(1000000)  FirstBitToTransfer=Most significant bit (MSB)  ClockMode=0  BlockFunction=Write  EnableRegisterAddress=on  RegisterAddress=0  OutputDataType=int8  OutputDataLength=1  BlockingMode=off  DataBits=16  UseCustomSSPin=Provided by the SPI peripheral  ActiveLowSSPin=Active low  Pin=0
      settings: SourceProductName=Embedded Coder Support Package for Texas Instruments C2000 Processors  SourceProductBaseCode=TIC2000
  Terminator : Terminator
  IrrLog : Outport
  wires:
  Constant/1 -> Mux/1
  SPI Transmit/1 -> Terminator/1
  Mux/1 -> SPI Transmit/1
  Irr/1 -> IrrLog/1, Mux/2

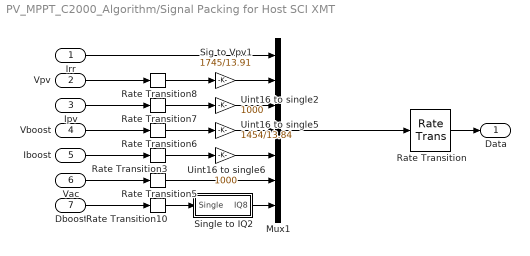
== system PV_MPPT_C2000_Algorithm/Signal Packing for Host SCI XMT ==
  Irr : Inport
  Vpv : Inport  Port=2
  Ipv : Inport  Port=3
  Vboost : Inport  Port=4
  Iboost : Inport  Port=5
  Vac : Inport  Port=6
  Dboost : Inport  Port=7
  Mux1 : Mux  Inputs=7
  Rate Transition{,3,5..8,10} (7 alike) : RateTransition  OutPortSampleTime=Tdata
  Sig to Vpv1 : Gain  Gain=1745/13.91  OutDataTypeStr=uint16
  Single to IQ2 : Subsystem
  Uint16 to single2 : Gain  Gain=1000  OutDataTypeStr=uint16
  Uint16 to single5 : Gain  Gain=1454/13.84  OutDataTypeStr=uint16
  Uint16 to single6 : Gain  Gain=1000  OutDataTypeStr=uint16
  Data : Outport
  wires:
  Mux1/1 -> Rate Transition/1
  Iboost/1 -> Rate Transition3/1
  Vac/1 -> Rate Transition5/1
  Vpv/1 -> Rate Transition8/1
  Vboost/1 -> Rate Transition6/1
  Rate Transition/1 -> Data/1
  Ipv/1 -> Rate Transition7/1
  Rate Transition5/1 -> Mux1/6
  Single to IQ2/1(IQ8) -> Mux1/7
  Uint16 to single6/1 -> Mux1/5
  Rate Transition7/1 -> Uint16 to single2/1
  Irr/1 -> Mux1/1
  Rate Transition3/1 -> Uint16 to single6/1
  Uint16 to single2/1 -> Mux1/3
  Rate Transition6/1 -> Uint16 to single5/1
  Sig to Vpv1/1 -> Mux1/2
  Uint16 to single5/1 -> Mux1/4
  Rate Transition8/1 -> Sig to Vpv1/1
  Rate Transition10/1 -> Single to IQ2/1(Single)
  Dboost/1 -> Rate Transition10/1

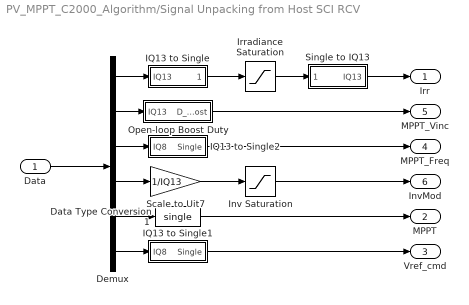
== system PV_MPPT_C2000_Algorithm/Signal Unpacking from Host SCI RCV ==
  Data : Inport
  Data Type Conversion1 : DataTypeConversion  OutDataTypeStr=single
  Demux : Demux  Outputs=6
  IQ13 to Single : Subsystem
  IQ13 to Single1 : Subsystem
  IQ13 to Single2 : Subsystem
  Inv Saturation : Saturate  UpperLimit=0.8  LowerLimit=0  OutDataTypeStr=Inherit: Inherit via back propagation  RndMeth=Simplest
  Irradiance Saturation : Saturate  UpperLimit=0.8  LowerLimit=0  OutDataTypeStr=Inherit: Inherit via back propagation  RndMeth=Simplest
  Open-loop Boost Duty : Subsystem
  Scale to Uit7 : Gain  Gain=1/IQ13  OutDataTypeStr=single
  Single to IQ13 : Subsystem
  Irr : Outport
  MPPT : Outport  Port=2
  Vref_cmd : Outport  Port=3
  MPPT_Freq : Outport  Port=4
  MPPT_Vinc : Outport  Port=5
  InvMod : Outport  Port=6
  wires:
  Data/1 -> Demux/1
  Inv Saturation/1 -> InvMod/1
  IQ13 to Single/1(Single) -> Irradiance Saturation/1
  Scale to Uit7/1 -> Inv Saturation/1
  Irradiance Saturation/1 -> Single to IQ13/1(Single)
  Demux/2 -> Open-loop Boost Duty/1(IQ13)
  Demux/1 -> IQ13 to Single/1(IQ13)
  Demux/4 -> Scale to Uit7/1
  Demux/3 -> IQ13 to Single2/1(IQ8)
  Single to IQ13/1(IQ13) -> Irr/1
  Open-loop Boost Duty/1(D_Boost) -> MPPT_Vinc/1
  Demux/5 -> Data Type Conversion1/1
  Demux/6 -> IQ13 to Single1/1(IQ8)
  IQ13 to Single1/1(Single) -> Vref_cmd/1
  Data Type Conversion1/1 -> MPPT/1
  IQ13 to Single2/1(Single) -> MPPT_Freq/1

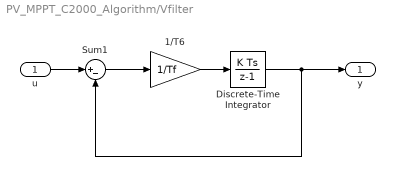
== system PV_MPPT_C2000_Algorithm/Vfilter ==
  u : Inport
  1/T6 : Gain  Gain=1/Tf
  Discrete-Time Integrator : DiscreteIntegrator  SampleTime=Tcontrol  ICPrevOutput=DiscIntNeverNeededParam  ICPrevScaledInput=DiscIntNeverNeededParam
  Sum1 : Sum  Inputs=|+-
  y : Outport
  wires:
  1/T6/1 -> Discrete-Time Integrator/1
  u/1 -> Sum1/1
  Discrete-Time Integrator/1 -> y/1, Sum1/2
  Sum1/1 -> 1/T6/1

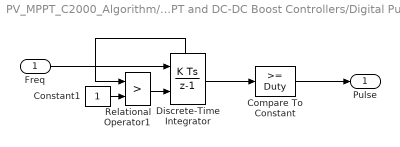
== system PV_MPPT_C2000_Algorithm/MPPT and DC-DC Boost Controllers/Digital Pulse ==
  Freq : Inport
  Compare To Constant : simulink/Logic and Bit Operations/Compare To Constant  relop=>=  const=Duty  OutDataTypeStr=boolean
  Constant1 : Constant
  Discrete-Time Integrator : DiscreteIntegrator  ExternalReset=rising  SampleTime=Ts  ShowStatePort=on  ICPrevOutput=DiscIntNeverNeededParam  ICPrevScaledInput=DiscIntNeverNeededParam
  Relational Operator1 : RelationalOperator  Operator=>  OutDataTypeStr=boolean  RndMeth=Nearest
  Pulse : Outport
  wires:
  Relational Operator1/1 -> Discrete-Time Integrator/2
  Constant1/1 -> Relational Operator1/2
  Compare To Constant/1 -> Pulse/1
  Discrete-Time Integrator/State -> Relational Operator1/1
  Discrete-Time Integrator/1 -> Compare To Constant/1
  Freq/1 -> Discrete-Time Integrator/1

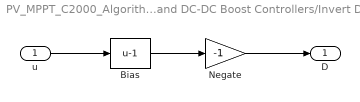
== system PV_MPPT_C2000_Algorithm/MPPT and DC-DC Boost Controllers/Invert Duty ==
  u : Inport
  Bias : Bias  Bias=-1
  Negate : Gain  Gain=-1  OutDataTypeStr=single
  D : Outport
  wires:
  Bias/1 -> Negate/1
  u/1 -> Bias/1
  Negate/1 -> D/1

== system PV_MPPT_C2000_Algorithm/Signal Packing for Host SCI XMT/Single to IQ2 ==
  Single : Inport
  Data Type Conversion : DataTypeConversion  OutDataTypeStr=uint16
  Scale to Uint16 : Gain  Gain=IQ8  OutDataTypeStr=single
  IQ8 : Outport
  wires:
  Data Type Conversion/1 -> IQ8/1
  Scale to Uint16/1 -> Data Type Conversion/1
  Single/1 -> Scale to Uint16/1

== system PV_MPPT_C2000_Algorithm/Signal Unpacking from Host SCI RCV/IQ13 to Single ==
  IQ13 : Inport
  Data Type Conversion1 : DataTypeConversion  OutDataTypeStr=single
  Remove IQ13 Scaling Uint : Gain  Gain=1/IQ13  OutDataTypeStr=single
  Single : Outport
  wires:
  Data Type Conversion1/1 -> Remove IQ13 Scaling Uint/1
  IQ13/1 -> Data Type Conversion1/1
  Remove IQ13 Scaling Uint/1 -> Single/1

== system PV_MPPT_C2000_Algorithm/Signal Unpacking from Host SCI RCV/IQ13 to Single1 ==
  IQ8 : Inport
  Data Type Conversion1 : DataTypeConversion  OutDataTypeStr=single
  Remove IQ8 Scaling Uint : Gain  Gain=1/IQ8  OutDataTypeStr=single
  Single : Outport
  wires:
  Data Type Conversion1/1 -> Remove IQ8 Scaling Uint/1
  IQ8/1 -> Data Type Conversion1/1
  Remove IQ8 Scaling Uint/1 -> Single/1

== system PV_MPPT_C2000_Algorithm/Signal Unpacking from Host SCI RCV/IQ13 to Single2 ==
  IQ8 : Inport
  Data Type Conversion1 : DataTypeConversion  OutDataTypeStr=single
  Remove IQ8 Scaling Uint : Gain  Gain=1/IQ8  OutDataTypeStr=single
  Single : Outport
  wires:
  Remove IQ8 Scaling Uint/1 -> Single/1
  IQ8/1 -> Data Type Conversion1/1
  Data Type Conversion1/1 -> Remove IQ8 Scaling Uint/1

== system PV_MPPT_C2000_Algorithm/Signal Unpacking from Host SCI RCV/Open-loop Boost Duty ==
  IQ13 : Inport
  Duty Saturation : Saturate  UpperLimit=0.9  LowerLimit=0  OutDataTypeStr=Inherit: Inherit via back propagation  RndMeth=Simplest
  Scale to Uint2 : Gain  Gain=1/IQ13  OutDataTypeStr=single
  D_Boost : Outport
  wires:
  IQ13/1 -> Scale to Uint2/1
  Scale to Uint2/1 -> Duty Saturation/1
  Duty Saturation/1 -> D_Boost/1

== system PV_MPPT_C2000_Algorithm/Signal Unpacking from Host SCI RCV/Single to IQ13 ==
  Single : Inport
  Data Type Conversion : DataTypeConversion  OutDataTypeStr=uint16
  Scale to Uint16 : Gain  Gain=IQ13  OutDataTypeStr=single
  IQ13 : Outport
  wires:
  Single/1 -> Scale to Uint16/1
  Scale to Uint16/1 -> Data Type Conversion/1
  Data Type Conversion/1 -> IQ13/1

== stateflow chart PV_MPPT_C2000_Algorithm/MPPT and DC-DC Boost Controllers/Perturb and Observe MPPT ==
  state DisableMPPT
    during:
    Vref = VrefCmd;
    Vref_prev = VrefCmd;
  state EnableMPPT
    state Compute_Power
      entry:
      P = V*I;
    state Calculate_Difference
      entry:
      deltaP = P - Pprev;
      deltaV = V - Vprev;
    state Decrement_Vref
      entry:
      Vref = Vref_prev - delV;
    state Increment_Vref
      entry:
      Vref = Vref_prev + delV;
    state Save_PreviousValues
      entry:
      Pprev = P; Vprev = V;
    state Clamp_VrefMax
      entry:
      Vref = VrefMax;
    state Clamp_VrefMin
      entry:
      Vref = VrefMin;
    (default) -> Compute_Power
    (junction 76) -> Compute_Power
    (junction 53) -> (junction 76) : {Vref_prev = Vref;}
    Compute_Power -> Calculate_Difference
    Calculate_Difference -> (junction 13) [order 1] : [deltaP < 0]
    Calculate_Difference -> (junction 14) [order 2] : [deltaP >= 0]
    (junction 13) -> Increment_Vref [order 2] : [deltaV < 0]
    (junction 14) -> Decrement_Vref [order 1] : [deltaV <= 0]
    (junction 13) -> Decrement_Vref [order 1] : [deltaV >= 0]
    (junction 14) -> Increment_Vref [order 2] : [deltaV > 0]
    Decrement_Vref -> Save_PreviousValues
    Increment_Vref -> Save_PreviousValues
    Save_PreviousValues -> (junction 53) [order 3]
    (junction 73) -> (junction 53)
    Save_PreviousValues -> Clamp_VrefMax [order 1] : [Vref >= VrefMax]
    Save_PreviousValues -> Clamp_VrefMin [order 2] : [Vref <= VrefMin]
    Clamp_VrefMax -> (junction 70)
    Clamp_VrefMin -> (junction 50)
    (junction 70) -> (junction 50)
    (junction 50) -> (junction 73)
  (default) -> DisableMPPT
  (junction 91) -> DisableMPPT
  EnableMPPT -> (junction 91) : [MPPT ~= 1]
  DisableMPPT -> EnableMPPT : [MPPT == 1]
  data: P local single =single(0); k local single =single(0); Psum local single =single(0); Vsum local single =single(0); Vavg local single =single(0); Pavg local single =single(0); deltaP local single =single(0); Pprev local single =single(0); Vprev local single =single(0); deltaV local single =single(0); Vref output single =single(5); Vref_prev local single =single(5); VrefMax constant single =single(10); VrefMin constant single =single(2); V input single; I input single; VrefCmd input single; MPPT input single; delV input single
  events: event input RISING_EDGE_EVENT
